simulink model "FIRP_Linear"  (R2021a)
settings: Solver=VariableStepAuto  StartTime=0.0  StopTime=50  RelTol=1e-6  AbsTol=1e-6
values from neighbouring files (symbols this model uses):
  K = -(place(A,B,p))    [ass_7.m]
  L = Gamma - K*PI    [ass_7.m]
  w = 10    [ass_7.m]
settings Model: Creator=simon  LastModifiedBy=simon

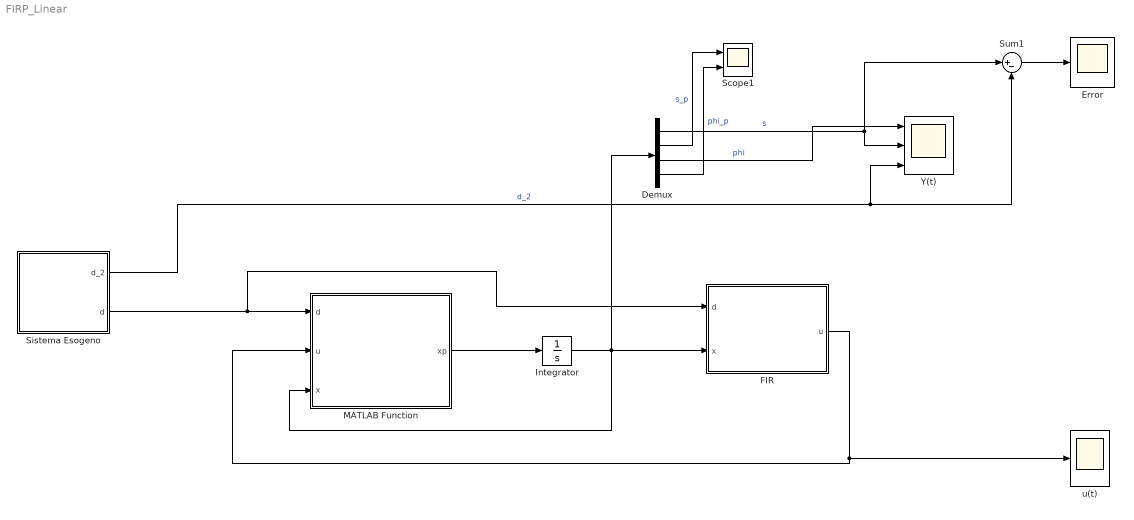
== system FIRP_Linear ==
  Demux : Demux
  Error : Scope
  FIR : Subsystem
  Integrator : Integrator
  MATLAB Function : MATLAB Function  TreatAsAtomicUnit=on
  Scope1 : Scope  NumInputPorts=2
  Sistema Esogeno : Subsystem
  Sum1 : Sum  Inputs=|+-
  Y(t) : Scope  NumInputPorts=3
  u(t) : Scope
  wires:
  MATLAB Function/1(xp) -> Integrator/1
  Integrator/1 -> MATLAB Function/3(x), FIR/2(x), Demux/1
  Demux/1 -> Y(t)/2, Sum1/1  "s"
  Sum1/1 -> Error/1
  Sistema Esogeno/1(d_2) -> Y(t)/3, Sum1/2  "d_2"
  Sistema Esogeno/2(d) -> FIR/1(d), MATLAB Function/1(d)
  Demux/3 -> Y(t)/1  "phi"
  Demux/2 -> Scope1/1  "s_p"
  Demux/4 -> Scope1/2  "phi_p"
  FIR/1(u) -> MATLAB Function/2(u), u(t)/1

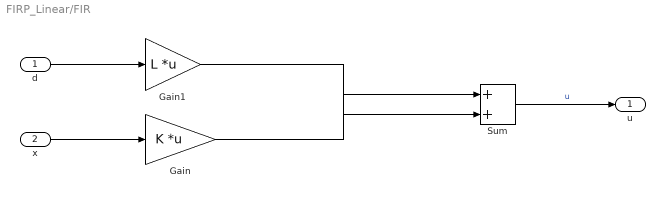
== system FIRP_Linear/FIR ==
  d : Inport
  x : Inport  Port=2
  Gain : Gain  Gain=K  Multiplication=Matrix(K*u)
  Gain1 : Gain  Gain=L  Multiplication=Matrix(K*u)
  Sum : Sum
  u : Outport
  wires:
  Gain1/1 -> Sum/2
  Sum/1 -> u/1  "u"
  Gain/1 -> Sum/1
  x/1 -> Gain/1
  d/1 -> Gain1/1

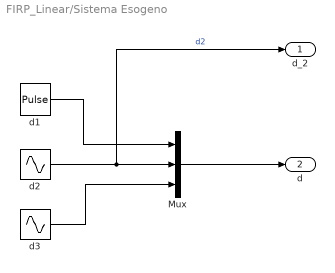
== system FIRP_Linear/Sistema Esogeno ==
  Mux : Mux  Inputs=3
  d1 : DiscretePulseGenerator  PulseType=Time based  Amplitude=0.5  Period=50  PulseWidth=50
  d2 : Sin  Frequency=w  SampleTime=0
  d3 : Sin  Frequency=w  Phase=pi/2  SampleTime=0
  d_2 : Outport
  d : Outport  Port=2
  wires:
  d3/1 -> Mux/3
  d2/1 -> d_2/1, Mux/2  "d2"
  d1/1 -> Mux/1
  Mux/1 -> d/1

== matlab function FIRP_Linear/MATLAB Function ==
  data: d input; u input; xp output; x input
function xp  = LinearizatedSpaceState(d,u,x)

M = 1;
F = 1;
l = 1;
g = 9.81;

xp = zeros(4,1); 

A = [0   1    0   0;
     0 -F/M   0   0;
     0   0    0   1;
     0 F/M*l g/l 0];

B = [0;1/M;0;-(1/M*l)];

% C = [1 0 0 0;
%      0 0 1 0];
 
P = [B zeros(4,1) zeros(4,1)]; 
% P altre due colonne nulle
%Pes = [P zeros(4,1) zeros(4,1)];

xp = A*x + B*u + P*d;
